simulink model "Wheel_Speed_System"  (R2020a)
settings: Solver=ode45  StartTime=0.0  StopTime=25  MaxStep=0.01  RelTol=1e-3  AbsTol=1e-6
model workspace (MAT data in the model file):
  I = 5
  Kf = 1
  PBmax = 1500
  Rr = 1.25
  TB = 0.01
  v0 = 44
settings Model: Creator=Noel Varghese  LastModifiedBy=Noel Varghese
settings DataIOCC: SaveOutput=off  SaveTime=off

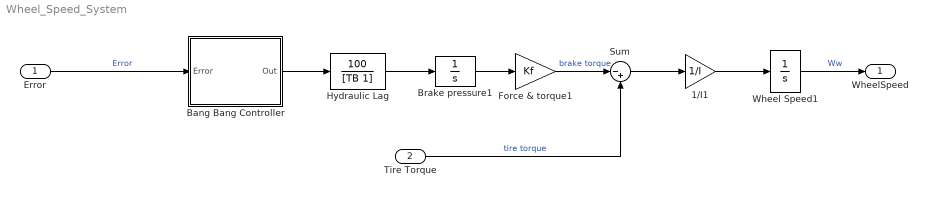
== system Wheel_Speed_System ==
  Error : Inport  OutDataTypeStr=double  PortDimensions=1  SampleTime=0
  Tire Torque : Inport  Port=2  OutDataTypeStr=double  PortDimensions=1  SampleTime=0
  1/I1 : Gain  Gain=1/I  SaturateOnIntegerOverflow=on  OutDataTypeStr=Inherit: Same as input  ParamDataTypeStr=Inherit: Same as input
  Bang Bang Controller : Subsystem
  Brake pressure1 : Integrator  LimitOutput=on  UpperSaturationLimit=PBmax  LowerSaturationLimit=0
  Force & torque1 : Gain  Gain=Kf  SaturateOnIntegerOverflow=on  OutDataTypeStr=Inherit: Same as input  ParamDataTypeStr=Inherit: Same as input
  "Hydraulic Lag " : TransferFcn  Numerator=[100]  Denominator=[TB 1]
  Sum : Sum  Inputs=|-+  InputSameDT=on  SaturateOnIntegerOverflow=on  OutDataTypeStr=Inherit: Same as first input
  Wheel Speed1 : Integrator  InitialCondition=v0/Rr  LimitOutput=on  UpperSaturationLimit=1000  LowerSaturationLimit=0
  WheelSpeed : Outport  OutDataTypeStr=double  PortDimensions=1  SampleTime=0  VectorParamsAs1DForOutWhenUnconnected=off
  wires:
  Error/1 -> Bang Bang Controller/1(Error)  "Error"
  Wheel Speed1/1 -> WheelSpeed/1  "Ww"
  1/I1/1 -> Wheel Speed1/1
  Force & torque1/1 -> Sum/1  "brake torque"
  "Hydraulic Lag "/1 -> Brake pressure1/1
  Brake pressure1/1 -> Force & torque1/1
  Tire Torque/1 -> Sum/2  "tire torque"
  Sum/1 -> 1/I1/1
  Bang Bang Controller/1(Out) -> "Hydraulic Lag "/1

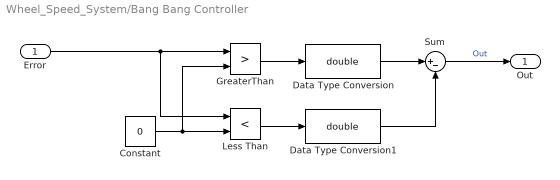
== system Wheel_Speed_System/Bang Bang Controller ==
  Error : Inport  SampleTime=0
  Constant : Constant  Value=0
  Data Type Conversion : DataTypeConversion  OutDataTypeStr=double  RndMeth=Zero
  Data Type Conversion1 : DataTypeConversion  OutDataTypeStr=double  RndMeth=Zero
  GreaterThan : RelationalOperator  Operator=>  OutDataTypeStr=boolean  RndMeth=Simplest
  Less Than : RelationalOperator  Operator=<  OutDataTypeStr=boolean  RndMeth=Simplest
  Sum : Sum  Inputs=|+-
  Out : Outport
  wires:
  Data Type Conversion/1 -> Sum/1
  Sum/1 -> Out/1  "Out"
  Less Than/1 -> Data Type Conversion1/1
  Constant/1 -> Less Than/2, GreaterThan/2
  Data Type Conversion1/1 -> Sum/2
  Error/1 -> GreaterThan/1, Less Than/1
  GreaterThan/1 -> Data Type Conversion/1
